simulink library "AtomicLibrary"  (Simulink 7.4)
settings: Solver=ode45  StartTime=0.0  StopTime=10.0  RelTol=1e-3
PostLoadFcn:
  | PacketBusGenerator
libraries: simulink x6, LinkLayer x5
(part 2 of 2)

== stateflow chart StrikeProcessing/StrikeProcessing_Statechart ==
  state chart
    state chartRegion [parallel]
      settings: executionOrder=2
      state Init
        state Receiving
          Receiving -> Receiving : [BAT_Info_checkQueue(EVT_TRANSFERBATINFO_POSX, BAT_InfoReadOut) && BAT_Info_checkQueue(EVT_TRANSFERBATINFO_POSY, BAT_InfoReadOut) && BAT_Info_checkQueue(EVT_TRANSFERBATINFO_POSZ, BAT_InfoReadOut) && BAT_Info_checkQueue(EVT_TRANSFERBATINFO_TIMEOFARRIVAL, BAT_InfoReadOut) && BAT_Info_checkQueue(EVT_TRANSFERBATINFO_VELOCITY, BAT_InfoReadOut)]
              | {[BAT_InfoReadOut, BAT_InfoParamReadOut, tmp_var_1] = BAT_Info_dequeue(EVT_TRANSFERBATINFO_POSX, BAT_InfoReadOut, BAT_InfoParamReadOut);
              | [BAT_InfoReadOut, BAT_InfoParamReadOut, tmp_var_2] = BAT_Info_dequeue(EVT_TRANSFERBATINFO_POSY, BAT_InfoReadOut, BAT_InfoParamReadOut);
              | [BAT_InfoReadOut, BAT_InfoParamReadOut, tmp_var_3] = BAT_Info_dequeue(EVT_TRANSFERBATINFO_POSZ, BAT_InfoReadOut, BAT_InfoParamReadOut);
              | [BAT_InfoReadOut, BAT_InfoParamReadOut, tmp_var_4] = BAT_Info_dequeue(EVT_TRANSFERBATINFO_TIMEOFARRIVAL, BAT_InfoReadOut, BAT_InfoParamReadOut);
              | [BAT_InfoReadOut, BAT_InfoParamReadOut, tmp_var_5] = BAT_Info_dequeue(EVT_TRANSFERBATINFO_VELOCITY, BAT_InfoReadOut, BAT_InfoParamReadOut); posX = tmp_var_1 ;  posY = tmp_var_2 ;  posZ = tmp_var_3 ;  timeOfArrival = tmp_var_4 ;  velocity = tmp_var_5 ; }
        (default) -> Receiving
      (default) -> Init
    state DataInit [parallel]
      settings: executionOrder=1
      DataInit -> DataInit : {BAT_InfoWriteOut = BAT_InfoWriteIn;
          | BAT_InfoParamWriteOut = BAT_InfoParamWriteIn;
          | BAT_InfoReadOut = BAT_InfoReadIn;
          | BAT_InfoParamReadOut = BAT_InfoParamReadIn;
          | ; }
  (default) -> chart
  data: posX local double; posY local double; posZ local double; timeOfArrival local double; velocity local double; clock function_input double; logicalTime function_output uint32; clock function_output double; event function_input uint8; evtQueueIn function_input uint8 size=[10,2]; param function_input double; paramQueueIn function_input double size=[10]; evtQueue function_output uint8 size=[10,2]; paramQueue function_output double size=[10]; event function_input uint8; evtQueueIn function_input uint8 size=[10,2]; paramQueueIn function_input double size=[10]; evtQueue function_output uint8 size=[10,2]; paramQueue function_output double size=[10]; parameter function_output double; event function_input uint8; evtQueue function_input uint8 size=[10,2]; available function_output boolean; clockSignal input double; BAT_InfoReadIn input uint8 size=[10,2]; BAT_InfoParamReadIn input double size=10; BAT_InfoWriteIn input uint8 size=[10,2]; BAT_InfoParamWriteIn input double size=10; BAT_InfoReadOut output uint8 size=[10,2]; BAT_InfoParamReadOut output double size=10; BAT_InfoWriteOut output uint8 size=[10,2]; BAT_InfoParamWriteOut output double size=10; EVT_TRANSFERBATINFO_POSX constant uint32 =6; EVT_TRANSFERBATINFO_POSY constant uint32 =7; EVT_TRANSFERBATINFO_POSZ constant uint32 =8; EVT_TRANSFERBATINFO_TIMEOFARRIVAL constant uint32 =9; EVT_TRANSFERBATINFO_VELOCITY constant uint32 =10; tmp_var_1 local double; tmp_var_2 local double; tmp_var_3 local double; tmp_var_4 local double; tmp_var_5 local double
  function logicalTime = time(clock):
    | function logicalTime = time(clock) 
    | 
    |  sample = 0.001;  % the sample time of the system clock 
    | 
    |  %convert to pass units of time after last reset 
    | 
    |  logicalTime = uint32((clockSignal - clock)/sample);
  function clock = reset():
    | function clock = reset() 
    | 
    |  %set clock variable to current time 
    | 
    |  clock = clockSignal;
  function [evtQueue, paramQueue] = BAT_Info_enqueue(event, evtQueueIn, param, paramQueueIn):
    | function [evtQueue, paramQueue] = BAT_Info_enqueue(event, evtQueueIn, param, paramQueueIn) %eml 
    |  evtQueue = evtQueueIn; 
    |  paramQueue = paramQueueIn; 
    |  for i = 1:length(evtQueue) 
    |  	if evtQueue(i) == uint8(0) 
    |  		evtQueue(i) = event; 
    |  		paramQueue(i) = param; 
    |  		return 
    |  	end 
    |  end
  function [evtQueue, paramQueue, parameter] = BAT_Info_dequeue(event, evtQueueIn, paramQueueIn):
    | function [evtQueue, paramQueue, parameter] = BAT_Info_dequeue(event, evtQueueIn, paramQueueIn) %eml 
    |   evtQueue = evtQueueIn; 
    |   paramQueue = paramQueueIn; 
    |   parameter = 0; 
    |   for i = 1:length(evtQueue) 
    |     if evtQueue(i) == event 
    |          parameter = paramQueue(i); 
    |          for j = i:length(evtQueue)-1 
    |              evtQueue(j) = evtQueue(j+1); 
    |              %Compatibility 
    |              evtQueue(j+length(evtQueue)) = evtQueue(j+1+length(evtQueue)); 
    |              paramQueue(j) = paramQueue(j+1); 
    |          end 
    |          evtQueue(length(evtQueue)) = 0; 
    |          %Compatibility 
    |          evtQueue(length(evtQueue)+length(evtQueue)) = 0; 
    |          paramQueue(length(paramQueue)) = 0; 
    |          return 
    |      end 
    |   end
  function available = BAT_Info_checkQueue(event, evtQueue):
    | function available = BAT_Info_checkQueue(event, evtQueue) %eml 
    |  available = false; 
    |  for i = 1:length(evtQueue) 
    |      if evtQueue(i) == event 
    |          available = true;    
    |          return 
    |      end 
    |  end
